simulink model "ATTN"  (R2023a)
settings: Solver=FixedStepAuto  StartTime=0.0  StopTime=40000  RelTol=1e-3
model workspace (MAT data in the model file):
  SampleTime = 0.001
  T_npxls = 4
  T_pupil = 100
  T_whisk = 20
  maxFrame = 3600000
  rewardDuration = 0.05
  targetSide = 1
  toneDuration = 1.5
  trainingStage = 3
  triangleAmplitude = 10
  triangleDuration = 0.1
undefined symbols (not defined in the file or in its folder): Ended, fdesignblkfcn, gcbh, Single
libraries: speedgoatlib_IO191 x5
(part 2 of 3)

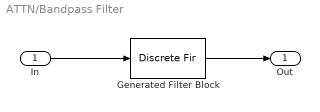
== system ATTN/Bandpass Filter ==
  In : Inport
  Generated Filter Block : DiscreteFir  Tag=BlockMethodSubSystem  FilterStructure=Direct form symmetric  Coefficients=[-2.4454897006896513e-06 -2.56742173651953851e-06 -2.6904861545531488e-06 -2.81454714397193635e-06 -2.93946535214558641e-06 -3.06509803031091609e-06 -3.19129918589820491e-06 -3.31791974136534052e-06 -3.44480769938805513e-06 -3.57180831424570957e-06 -3.6987642692300706e-06 -3.8255158598941323e-06 -3.9519011829499759e-06 -4.07775633061091228e-06 -4.20291559016737714e-06 -4.32721164857290318e-06 -4.45047580180991913e-06 -4.57253816879339651e-06 -4.69322790956374843e-06 -4.8123734475098501e-06 -4.92980269535605193e-06 -5.04534328463753935e-06 -5.15882279838227398e-06 -5.27006900670890746e-06 -5.37891010504324102e-06 -5.48517495464968105e-06 -5.58869332516680343e-06 -5.68929613883073187e-06 -5.78681571606370287e-06 -5.88108602210100086e-06 -5.97194291432307867e-06 -6.05922438995672689e-06 -6.14277083380392516e-06 -6.22242526565437995e-06 -6.29803358703354215e-06 -6.36944482693648908e-06 -6.43651138619465127e-06 -6.49908928012128943e-06 -6.55703837908017639e-06 -6.61022264662100308e-06 -6.6585103748249614e-06 -6.70177441650380619e-06 -6.73989241389677914e-06 -6.77274702351052664e-06 -6.80022613674919182e-06 -6.82222309598376366e-06 -6.83863690571265582e-06 -6.84937243846851868e-06 -6.85434063513022441e-06 -6.8534586993027498e-06 -6.84665028543312436e-06 -6.83384568033498058e-06 -6.81498197780058264e-06 -6.79000324598519844e-06 -6.7588606872556066e-06 -6.7215127902011652e-06 -6.6779254735145738e-06 -6.62807222145621961e-06 -6.57193421062661881e-06 -6.50950042777781941e-06 -6.44076777840752028e-06 -6.36574118588637646e-06 -6.28443368088219129e-06 -6.19686648085330975e-06 -6.10306905939659581e-06 -6.00307920524582762e-06 -5.89694307072888454e-06 -5.78471520950516905e-06 -5.66645860341573113e-06 -5.54224467829441058e-06 -5.41215330859853472e-06 -5.27627281073555752e-06 -5.13469992497098551e-06 -4.98753978582351413e-06 -4.83490588086176477e-06 -4.67691999783725106e-06 -4.51371216009933806e-06 -4.34542055025563724e-06 -4.17219142205730692e-06 -3.99417900050058786e-06 -3.81154537015837133e-06 -3.62446035176441086e-06 -3.43310136709531978e-06 -3.23765329220624862e-06 -3.03830829909817188e-06 -2.83526568590412352e-06 -2.62873169570644138e-06 -2.41891932410507237e-06 -2.20604811568059974e-06 -1.99034394950661538e-06 -1.77203881388551769e-06 -1.55137057049779708e-06 -1.32858270816880078e-06 -1.10392408647583881e-06 -8.77648669431910269e-07 -6.50015249500740855e-07 -4.21287162209172574e-07 -1.91731991643504118e-07 3.83787328738238149e-08 2.68769848611957874e-07 4.99162879436978308e-07 7.29276363651105298e-07 9.58826189311450054e-07 1.18752593665789316e-06 1.41508722726677149e-06 1.64122007953655106e-06 1.86563327009644334e-06 2.08803470071945437e-06 2.30813177030736605e-06 2.5256317515079827e-06 2.7402421715097328e-06 2.95167119655339559e-06 3.15962801968779996e-06 3.36382325128986446e-06 3.56396931185877859e-06 3.7597808265890518e-06 3.95097502121797448e-06 4.13727211863640978e-06 4.31839573574811592e-06 4.49407328005482627e-06 4.66403634544175454e-06 4.82802110663231549e-06 4.98576871178017947e-06 5.13702567266087042e-06 5.28154425192639895e-06 5.4190828468827203e-06 5.54940636925090163e-06 5.67228662037188987e-06 5.7875026613169812e-06 5.8948411773662372e-06 5.99409683632077295e-06 6.08507264011719913e-06 6.1675802692164393e-06 6.24144041924405756e-06 6.30648312936384278e-06 6.36254810187336759e-06 6.40948501251614932e-06 6.44715381101293179e-06 6.47542501132312705e-06 6.49417997115539655e-06 6.50331116025755296e-06 6.50272241702466551e-06 6.49232919297680992e-06 6.47205878466845959e-06 6.4418505526048911e-06 6.4016561267535234e-06 6.35143959825205895e-06 6.29117769693003751e-06 6.22085995427479805e-06 6.1404888514893769e-06 6.0500799523051377e-06 5.9496620202302234e-06 5.83927711993068915e-06 5.71898070246055245e-06 5.58884167407495812e-06 5.44894244837969805e-06 5.29937898158983258e-06 5.14026079069042842e-06 4.97171095431314121e-06 4.79386609616151712e-06 4.60687635084247577e-06 4.41090531197944271e-06 4.20612996250760769e-06 ...(+93727 chars)]  InputProcessing=Columns as channels (frame based)
  Out : Outport  VectorParamsAs1DForOutWhenUnconnected=off
  wires:
  In/1 -> Generated Filter Block/1
  Generated Filter Block/1 -> Out/1
